simulink library "powerlib"  (Simulink 6.0)
settings: Solver=ode45  SolverMode=SingleTasking  StartTime=0.0  StopTime=10.0  RelTol=1e-3
undefined symbols (not defined in the file or in its folder): com, ctrl1, Da, DiscIntNeverNeededParam, dtha, etat, FA, find_system, Ha, j, Ka, Ki, Kv, q0, Rground, sel, st_a, st_b, st_c, sta, stb, stc, T1, T2, T3, T4
libraries: powerlib_models x30, powerlib x25, simulink_extras x6, powerlib_extras x3, simulink x2
(part 4 of 7)

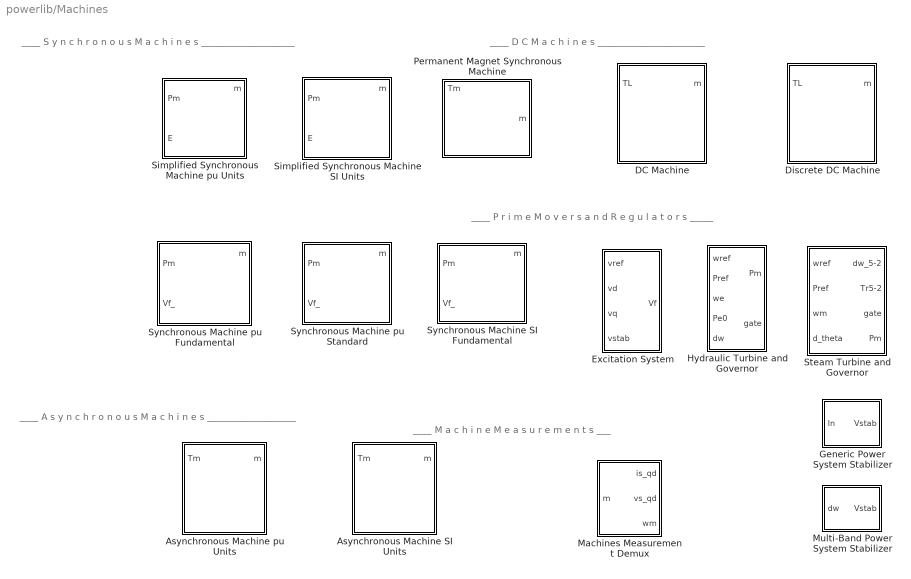
== system powerlib/Machines ==
  note: ____ A s y n c h r o n o u s M a c h i n e s ___________________
  note: ____ M a c h i n e M e a s u r e m e n t s ___
  note: ____ P r i m e M o v e r s a n d R e g u l a t o r s _____
  note: ____ D C M a c h i n e s _______________________
  note: ____ S y n c h r o n o u s M a c h i n e s ____________________
  Asynchronous Machine SI Units : Subsystem  mask(Asynchronous Machine){PresetModel=No, ShowDetailedParameters=on, RotorType=Wound, ReferenceFrame=Rotor, NominalParameters=[3730 460 60], Stator=[1.115 0.005974], Rotor=[1.083 0.005974], Lm=0.2037, Mechanical=[0.02 0.005752 2], InitialConditions=[ 1,0   0,0,0   0,0,0 ], Units=1, LoadFlowParameters=0}
      mask prompts: PresetModel "Preset model:"; ShowDetailedParameters "-----------------  Show detailed parameters -----------------"; RotorType "Rotor type:"; ReferenceFrame "Reference frame:"; NominalParameters "Nominal power, voltage (line-line), and frequency [ Pn(VA),Vn(Vrms),fn(Hz) ]:"; Stator "Stator resistance and inductance[ Rs(ohm)  Lls(H) ]:"; Rotor "Rotor resistance and inductance [ Rr'(ohm)  Llr'(H) ]:"; Lm "Mutual inductance Lm (H):"; Mechanical "Inertia, friction factor and pairs of poles [ J(kg.m^2)  F(N.m.s)  p() ]:"; InitialConditions "Initial conditions"; Units "IOunits"; LoadFlowParameters "Load flow Parameters"
      mask help:
      | Implements a three-phase asynchronous machine (wound rotor or squirrel cage)
      | modeled in the dq rotor reference frame. Stator and rotor windings are connected
      | in wye to an internal neutral point. You can specify initial values for stator and rotor
      | currents or for  the stator current only.
      mask init:
      | block = gcb;
      | ctrl = ReferenceFrame;
      | one_third=1/3; 
      | sqrt3_3=sqrt(3)/3;
      | sqrt3=sqrt(3);
      | switch RotorType
      |     case 1, selWidth=6; elements1=3:6; elements2=1:4;
      |     case 2, selWidth=4; elements1=1:4; elements2=3:4;
      | end
      | powericon('psbloadfunction',block,'gotofrom','Initialize');
      | [NominalParameters,Stator,Rotor,Lm,Mechanical,InitialConditions] = powericon('AsynchronousMachineConvert',NominalParameters,Stator,Rotor,Lm,Mechanical,InitialConditions);	
      | Ts = powericon('AsynchronousMachineInit',block);
      | [p1,p2,p3,p4,p5,p6,p7,p8,p9,p10,p11,p12,p13,p14,p15,p16] = powericon('AsynchronousMachineIcon');
      | [Rs,Lls,Rr,Llr,H,F,p,Laq,Lad,web_psb,Vb,Vb2,ib,ib2,phib2,Nb2,Tb2,phisqo,phisdo,phirqo,phirdo,wmo,tho] = powericon('AsynchronousMachineParam',NominalParameters,Stator,Rotor,Lm,Mechanical,InitialConditions,Units);
      | powericon('AsynchronousMachineCback',block);
      settings: CopyFcn=powericon('psbloadfunction',gcbh,'gotofrom','UpdateGotoTag');
      mask Help: web(psbhelp);
      mask StyleString: popup(No|01:  5 HP   460 V 60Hz 1750 RPM           |02:  10 HP  460 V 60Hz 1760 RPM          |03:  20 HP  460 V 60Hz 1760 RPM          |04:  50 HP  460 V 60Hz 1780 RPM          |05:  100 HP 460 V 60Hz 1780 RPM         |06:  150 HP 460 V 60Hz 1785 RPM         |07:  200 HP 460 V 60Hz 1785 RPM         |08:  5 HP   575 V 60Hz 1750 RPM           |09:  10 HP  575 V 60Hz 1760 RPM          |10:  20 HP  575 V 60Hz 1765 RPM          |11:  50 HP  575 V 60Hz 1775 RPM          |12:  100 HP 575 V 60Hz 1780 RPM         |13:  150 HP 575 V 60Hz 1785 RPM         |14:  200 HP 575 V 60Hz 1785 RPM         |15:  5.4 HP (4KW)   400 V  50Hz 1430 RPM  |16:  10 HP (7.5KW)  400 V 50Hz 1440 RPM |17:  20 HP (15KW)   400 V 50Hz 1460 RPM  |18:  50 HP (37KW)   400 V 50Hz 1480 RPM  |19:  100 HP (75KW)  400 V 50Hz 1484 RPM |20:  150 HP (110KW) 400 V 50Hz 1487 RPM|21:  215 HP (160KW) 400 V 50Hz 1487 RPM),checkbox,popup(Wound|Squirrel-cage),popup(Rotor|Stationary|Synchronous),edit,edit,edit,edit,edit,edit,edit,edit
      mask CallbackString: powericon('AsynchronousMachineCback',gcb,'SI');|powericon('AsynchronousMachineCback',gcb);|powericon('AsynchronousMachineCback',gcb);|||||||||
      mask Display: plot(-55,-30,55,90,p1,p2,p3,p4,p5,p6,p7,p8,p9,p10,p11,p12,p13,p14,p15,p16);color('blue');plot([-30,-10,-10],[70,70,55]);plot([35,10,10],[70,70,55]);
  Asynchronous Machine pu Units : Subsystem  mask(Asynchronous Machine){PresetModel=No, ShowDetailedParameters=on, RotorType=Wound, ReferenceFrame=Rotor, NominalParameters=[3730 460 60], Stator=[0.01965 0.0397], Rotor=[0.01909 0.0397], Lm=1.354, Mechanical=[0.09526 0.05479 2], InitialConditions=[ 1,0   0,0,0   0,0,0 ], Units=0, LoadFlowParameters=0}
      mask prompts: PresetModel "Preset model:"; ShowDetailedParameters "-----------------  Show detailed parameters -----------------"; RotorType "Rotor type:"; ReferenceFrame "Reference frame:"; NominalParameters "Nominal power, voltage (line-line), and frequency  [ Pn(VA),Vn(Vrms),fn(Hz) ]:"; Stator "Stator resistance and inductance  [ Rs,Lls ] (pu):"; Rotor "Rotor resistance and inductance  [ Rr',Llr' ] (pu):"; Lm "Mutual inductance Lm (pu):"; Mechanical "Inertia constant, friction factor and pairs of poles [ H(s) F(pu) p() ]:"; InitialConditions "Initial conditions"; Units "IOunits"; LoadFlowParameters "Load Flow Parameters"
      mask help:
      | Implements a three-phase asynchronous machine (wound rotor or squirrel cage)
      | modeled in the dq rotor reference frame. Stator and rotor windings are connected
      | in wye to an internal neutral point. You can specify initial values for stator and rotor
      | currents or for  the stator current only.
      mask init:
      | block = gcb;
      | ctrl = ReferenceFrame;
      | one_third=1/3; 
      | sqrt3_3=sqrt(3)/3;
      | sqrt3=sqrt(3);
      | switch RotorType
      |     case 1, selWidth=6; elements1=3:6; elements2=1:4;
      |     case 2, selWidth=4; elements1=1:4; elements2=3:4;
      | end
      | Ts = powericon('AsynchronousMachineInit',block);
      | powericon('psbloadfunction',block,'gotofrom','Initialize');
      | [p1,p2,p3,p4,p5,p6,p7,p8,p9,p10,p11,p12,p13,p14,p15,p16] = powericon('AsynchronousMachineIcon');
      | [Rs,Lls,Rr,Llr,H,F,p,Laq,Lad,web_psb,Vb,Vb2,ib,ib2,phib2,Nb2,Tb2,phisqo,phisdo,phirqo,phirdo,wmo,tho] = powericon('AsynchronousMachineParam',NominalParameters,Stator,Rotor,Lm,Mechanical,InitialConditions,Units);
      | powericon('AsynchronousMachineCback',block);
      settings: CopyFcn=powericon('psbloadfunction',gcb,'gotofrom','UpdateGotoTag');
      mask Help: web(psbhelp);
      mask StyleString: popup(No|01:  5 HP   460 V 60Hz 1750 RPM           |02:  10 HP  460 V 60Hz 1760 RPM          |03:  20 HP  460 V 60Hz 1760 RPM          |04:  50 HP  460 V 60Hz 1780 RPM          |05:  100 HP 460 V 60Hz 1780 RPM         |06:  150 HP 460 V 60Hz 1785 RPM         |07:  200 HP 460 V 60Hz 1785 RPM         |08:  5 HP   575 V 60Hz 1750 RPM           |09:  10 HP  575 V 60Hz 1760 RPM          |10:  20 HP  575 V 60Hz 1765 RPM          |11:  50 HP  575 V 60Hz 1775 RPM          |12:  100 HP 575 V 60Hz 1780 RPM         |13:  150 HP 575 V 60Hz 1785 RPM         |14:  200 HP 575 V 60Hz 1785 RPM         |15:  5.4 HP (4KW)   400 V  50Hz 1430 RPM  |16:  10 HP (7.5KW)  400 V 50Hz 1440 RPM |17:  20 HP (15KW)   400 V 50Hz 1460 RPM  |18:  50 HP (37KW)   400 V 50Hz 1480 RPM  |19:  100 HP (75KW)  400 V 50Hz 1484 RPM |20:  150 HP (110KW) 400 V 50Hz 1487 RPM|21:  215 HP (160KW) 400 V 50Hz 1487 RPM),checkbox,popup(Wound|Squirrel-cage),popup(Rotor|Stationary|Synchronous),edit,edit,edit,edit,edit,edit,edit,edit
      mask CallbackString: powericon('AsynchronousMachineCback',gcb,'pu');|powericon('AsynchronousMachineCback',gcb);|powericon('AsynchronousMachineCback',gcb);|||||||||
      mask Display: plot(-55,-30,55,90,p1,p2,p3,p4,p5,p6,p7,p8,p9,p10,p11,p12,p13,p14,p15,p16);color('blue');plot([-30,-10,-10],[70,70,55]);plot([35,10,10],[70,70,55]);
  DC Machine : Subsystem  LoadFcn=find_system(gcs,'FollowLinks', 'on', 'LookUnderMasks', 'all');  mask(DC machine){PresetModel=No, ShowDetailedParameters=on, RLa=[ 0.5  0.01], RLf=[ 240  120], Laf=1.8, J=0.05, Bm=0.02, Tf=0, w0=0}
      mask prompts: PresetModel "Preset  model"; ShowDetailedParameters "-----------------  Show detailed parameters -----------------"; RLa "Armature resistance and inductance [Ra (ohms) La (H) ]"; RLf "Field resistance and inductance [Rf (ohms) Lf (H) ]"; Laf "Field-armature mutual inductance Laf (H) :"; J "Total inertia J (kg.m^2)"; Bm "Viscous friction coefficient Bm (N.m.s)"; Tf "Coulomb friction torque Tf (N.m)"; w0 "Initial speed (rad/s) :"
      mask help: This block implements a separately excited DC machine. Access is provided to the field connections so that the machine can be used as a shunt-connected or a series-connected DC machine.
      mask init:
      | Ra=RLa(1); La=RLa(2);
      | 
      | Rf=RLf(1); Lf=RLf(2);
      mask Help: web(psbhelp)
      mask StyleString: popup(No|01: 5HP 240V 1750RPM Field:300V|02: 5HP 240V 1750RPM Field:150V|03: 5HP 500V 1750RPM Field:300V|04: 10HP 240V 1750RPM Field:300V|05: 10HP 500V 1750RPM Field:300V|06: 20HP 240V 1750RPM Field:300V|07: 20HP 500V 1750RPM Field:300V|08: 30HP 240V 1750RPM Field:300V|09: 30HP 500V 1750RPM Field:300V|10: 40HP 240V 1750RPM Field:300V|11: 40HP 500V 1750RPM Field:300V|12: 50HP 240V 1750RPM Field:300V|13: 50HP 500V 1750RPM Field:300V|14: 75HP 500V 1750RPM Field:300V|15: 100HP 500V 1750RPM Field:300V|16: 125HP 500V 1750RPM Field:300V|17: 150HP 500V 1750RPM Field:300V|18: 175HP 500V 1750RPM Field:300V|19: 200HP 440V 1184RPM Field:310V|20: 200HP 500V 1750RPM Field:150V|21: 200HP 500V 1750RPM Field:300V|22: 225HP 500V 1750RPM Field:300V|23: 250HP 500V 1750RPM Field:300V),checkbox,edit,edit,edit,edit,edit,edit,edit
      mask CallbackString: powericon('DCMachineCback',gcb,'Continuous');|powericon('DCMachineCback',gcb,'Continuous');|||||||
      mask Display:
      | plot(-80,-80,80,80,[0,9,18,24,29,30,29,24,18,9,0,-9,-18,-24,-29,-30,-29,-24,-18,-9,0],[30,29,24,18,9,0,-9,-18,-24,-29,-30,-29,-24,-18,-9,0,9,18,24,29,30],[-29,-35,-35,-29],[-8,-8,8,8],[29,35,35,29],[-8,-8,8,8],[-35,-55],[0,0],[35,55],[0,0],[-78,-50,-50,-49,-45,-39,-33,-26,-21,-18,-17,-19,-22,-22,-26,-27,-25,-22,-16,-9,-3,2,6,6,4,1,1,-3,-4,-2,2,7,14,20,26,29,30,28,24,24,21,20,21,25,31,37,44,49,50,50,50,78]*.7,[58,58,57.2,49.2,42.8,38.8,38,39.6,44.4,51.6,59.6,67.6,72.4,72.4,65.2,57.2,49.2,42.8,38.8,38,39.6,44.4,51.6,59.6,67.6,72.4,72.4,65.2,57.2,49.2,42.8,38.8,38,39.6,44.4,51.6,59.6,67.6,72.4,72.4,65.2,57.2,49.2,42.8,38.8,38,39.6,44.4,51.6,58,58,58]*.6-85 );
      | 
      | disp('dc')
      | 
      | color('blue');
      | 
      | plot([-50,-10,-10],[50,50,30]);
      | 
      | plot([50,10,10],[50,50,30]);
  Discrete DC Machine : Subsystem  LoadFcn=find_system(gcs,'FollowLinks', 'on', 'LookUnderMasks', 'all');  mask(Discrete DC machine){PresetModel=No, ShowDetailedParameters=on, RLa=[0.5  0.01], RLf=[240  120], Laf=1.8, J=0.05, Bm=0.02, Tf=0, w0=0, Ts=50e-6}
      mask prompts: PresetModel "Preset  model"; ShowDetailedParameters "-----------------  Show detailed parameters -----------------"; RLa "Armature resistance and inductance [Ra (ohms) La (H) ]"; RLf "Field resistance and inductance [Rf (ohms) Lf (H) ]"; Laf "Field-armature mutual inductance Laf (H) :"; J "Total inertia J (kg.m^2)"; Bm "Viscous friction coefficient Bm (N.m.s)"; Tf "Coulomb friction torque Tf (N.m)"; w0 "Initial speed (rad/s) :"; Ts "Sample Time"
      mask help: This block implements a separately excited DC machine. Access is provided to the field connections so that the machine can be used as a shunt-connected or a series-connected DC machine.
      mask init:
      | Ra=RLa(1); La=RLa(2);
      | 
      | Rf=RLf(1); Lf=RLf(2);
      settings: AttributesFormatString=\n
      mask Help: web(psbhelp)
      mask StyleString: popup(No|01: 5HP 240V 1750RPM Field:300V|02: 5HP 240V 1750RPM Field:150V|03: 5HP 500V 1750RPM Field:300V|04: 10HP 240V 1750RPM Field:300V|05: 10HP 500V 1750RPM Field:300V|06: 20HP 240V 1750RPM Field:300V|07: 20HP 500V 1750RPM Field:300V|08: 30HP 240V 1750RPM Field:300V|09: 30HP 500V 1750RPM Field:300V|10: 40HP 240V 1750RPM Field:300V|11: 40HP 500V 1750RPM Field:300V|12: 50HP 240V 1750RPM Field:300V|13: 50HP 500V 1750RPM Field:300V|14: 75HP 500V 1750RPM Field:300V|15: 100HP 500V 1750RPM Field:300V|16: 125HP 500V 1750RPM Field:300V|17: 150HP 500V 1750RPM Field:300V|18: 175HP 500V 1750RPM Field:300V|19: 200HP 440V 1184RPM Field:310V|20: 200HP 500V 1750RPM Field:150V|21: 200HP 500V 1750RPM Field:300V|22: 225HP 500V 1750RPM Field:300V|23: 250HP 500V 1750RPM Field:300V),checkbox,edit,edit,edit,edit,edit,edit,edit,edit
      mask CallbackString: powericon('DCMachineCback',gcb,'Discrete');|powericon('DCMachineCback',gcb,'Discrete');||||||||
      mask Display:
      | plot(-80,-80,80,80,[0,9,18,24,29,30,29,24,18,9,0,-9,-18,-24,-29,-30,-29,-24,-18,-9,0],[30,29,24,18,9,0,-9,-18,-24,-29,-30,-29,-24,-18,-9,0,9,18,24,29,30],[-29,-35,-35,-29],[-8,-8,8,8],[29,35,35,29],[-8,-8,8,8],[-35,-55],[0,0],[35,55],[0,0],[-78,-50,-50,-49,-45,-39,-33,-26,-21,-18,-17,-19,-22,-22,-26,-27,-25,-22,-16,-9,-3,2,6,6,4,1,1,-3,-4,-2,2,7,14,20,26,29,30,28,24,24,21,20,21,25,31,37,44,49,50,50,50,78]*.7,[58,58,57.2,49.2,42.8,38.8,38,39.6,44.4,51.6,59.6,67.6,72.4,72.4,65.2,57.2,49.2,42.8,38.8,38,39.6,44.4,51.6,59.6,67.6,72.4,72.4,65.2,57.2,49.2,42.8,38.8,38,39.6,44.4,51.6,59.6,67.6,72.4,72.4,65.2,57.2,49.2,42.8,38.8,38,39.6,44.4,51.6,58,58,58]*.6-85 );
      | 
      | disp('dc')
      | 
      | color('blue');
      | 
      | plot([-50,-10,-10],[50,50,30]);
      | 
      | plot([50,10,10],[50,50,30]);
  Excitation System : Subsystem  mask(Excitation System){tr=20e-3, reg=[ 300, 0.001 ], exc=[ 1, 0 ], tgr=[ 0, 0 ], damp=[ 0.001, 0.1 ], sat=[ 0, 0 ], lim=[ -11.5, 11.5, 0 ], v0=[1.0  1.28]}
      mask prompts: tr "Low-pass filter time constant Tr(s):"; reg "Regulator gain and time constant [ Ka()  Ta(s) ]:"; exc "Exciter  [ Ke()  Te(s) ]:"; tgr "Transient gain reduction [ Tb(s)  Tc(s) ]:"; damp "Damping filter gain and time constant  [ Kf()  Tf(s)  ]:"; sat "Field saturation parameters [ A, B ]:"; lim "Regulator output limits and gain [ Efmin, Efmax (p.u.), Kp() ]:"; v0 "Initial values of terminal voltage  and field voltage [ Vt0 (pu) Vf0(pu) ] :"
      mask help:
      | Implements an IEEE type 1 synchronous machine voltage regulator combined
      | to an exciter.
      |
      | The output of the block is the field voltage vfd, in p.u.,  to be applied to the Vf
      | Simulink input of a Synchronous Machine block.
      |
      | Connect the Vd and Vq measurements signals of the Synchronous Machine block
      | (signals 9 and 10)  to  the Vd and Vq inputs of the Excitation System block.
      mask init:
      | ka=reg(1);ta=reg(2);ke=exc(1);te=exc(2);tb=tgr(1);tc=tgr(2);kf=damp(1);tf=damp(2);efmin=lim(1);efmax=lim(2);a=sat(1);b=sat(2);kp=lim(3);
      | powericon('psbcallbacks',gcb,'Excitationsystem',1);
      mask Help: web(psbhelp);
  Generic Power System Stabilizer : Subsystem  mask(Generic Power System Stabilizer){Tsensor=30e-3, K=20, Twashout=2, Tleadlag1=[50e-3 20e-3], Tleadlag2=[3 5.4], VSlimits=[-0.15 0.15], Vinit=0, Plot_On=off, MagdB_On=on, FreqRange=logspace(-2,2,500)}
      mask prompts: Tsensor "Sensor time constant:"; K "Gain:"; Twashout "Wash-out time constant:"; Tleadlag1 "Lead-lag #1 time constants: [ Tnum Tden ]"; Tleadlag2 "Leag-lag #2 time constants: [ Tnum Tden ]"; VSlimits "Output limits: [ VSmin VSmax ]"; Vinit "Initial input:"; Plot_On "Plot frequency response"; MagdB_On "Magnitude in dB"; FreqRange "Frequency range (Hz):"
      mask help:
      | This block implements a generic Power System Stabilizer (PSS). It consists of a
      | low-pass filter, a general gain, a washout high-pass filter, a phase-compensation
      | system, and an output limiter.
      |
      | The input is the synchronous machine speed deviation with respect to nominal
      | (dw in pu) or the acceleration power (Pa=Pm-Pe in pu).
      |
      | The output is the stabilization voltage, in p.u.
      mask init:
      | powericon('psbcallbacks',gcb,'PSS',1);
      | T1n=Tleadlag1(1);
      | T1d=Tleadlag1(2);
      | T2n=Tleadlag2(1);
      | T2d=Tleadlag2(2);
      | %
      | if Plot_On==1,
      | % Compute global system (sysG):
      | numS=[1];
      | denS=[Tsensor 1];
      | sysS=tf(numS,denS);
      | numW=[Twashout 0];
      | denW=[Twashout 1];
      | sysW=tf(numW,denW);
      | numL1=[T1n 1];
      | denL1=[T1d 1];
      | sysL1=tf(numL1,denL1);
      | numL2=[T2n 1];
      | denL2=[T2d 1];
      | sysL2=tf(numL2,denL2);
      | sysG=sysS*K*sysW*sysL1*sysL2;
      | %
      | % Plot response:
      | w=2*pi*FreqRange;
      | [Mag,Pha]=bode(sysG,w);
      | subplot(2,1,1)
      | if  MagdB_On==1,
      | Y= 20*log10(squeeze(Mag)) ;
      | strLabel='dB';
      | else
      | Y=squeeze(Mag);
      | strLabel='pu/pu';
      | end
      | %
      | semilogx(FreqRange,Y)
      | ylabel(strLabel);grid;
      | title('PSS Frequency Response');
      | subplot(2,1,2);
      | semilogx(FreqRange,rem(squeeze(Pha),360))
      | ylabel('Degrees');grid;
      | xlabel('Frequency (Hz)');
      | end
      mask Help: web(psbhelp)
      mask CallbackString: |||||||powericon('psbcallbacks',gcbh,'PSSmodel');||
  Hydraulic Turbine and Governor : Subsystem  mask(Hydraulic Turbine and Governor){sm=[ 10/3  0.07 ], gate=[  0.01  0.97518  -0.1  0.1 ], reg=[  0.05  1.163  0.105  0  0.01  ], hyd=[  0  2.67  ], dref=0, po=0.7516}
      mask prompts: sm "Servo-motor [ Ka()  Ta(sec) ]:"; gate "Gate opening limits [ gmin,gmax(pu)    vgmin,vgmax(pu/s) ]:"; reg "Permanent droop and regulator  [ Rp() Kp() Ki() Kd() Td(s) ]:"; hyd "Hydraulic turbine [ beta()  Tw(sec) ]:"; dref "Droop reference (0=power error, 1=gate opening):"; po "Initial mechanical power (pu):"
      mask help: Implements a hydraulic turbine combined to a PID governor system.
      mask init:
      | ka=sm(1);ta=sm(2);gmin=gate(1);gmax=gate(2);vgmin=gate(3);vgmax=gate(4);Rp=reg(1);kp=reg(2);ki=reg(3);kd=reg(4);td=reg(5);beta=hyd(1);tw=hyd(2);go=po*(gmax-gmin);
      | powericon('psbcallbacks',gcb,'HTGsystem',1);
      mask Help: web(psbhelp);
  Machines Measurement Demux : Subsystem  mask(Machine measurements){machType=Synchronous, ssm1=on, ssm2=on, ssm3=on, ssm4=on, ssm5=on, ssm6=on, sm1=off, sm2=on, sm3=off, sm4=off, sm5=off, sm6=on, sm7=off, sm8=on, sm9=off, sm10=off, sm11=off, sm115=off, sm12=off, sm13=off, sm14=off, asm1=on, asm2=on, asm3=on, asm4=on, asm5=on, asm6=on, asm7=on, asm8=on, asm9=on, asm10=on, asm11=on, pmsm1=on, pmsm2=on, pmsm3=on, pmsm4=on, pmsm5=on, pmsm6=on, lastType=1}
      mask prompts: machType "Machine type:"; ssm1 "Line currents          [ isa  isb  isc ]"; ssm2 "Terminal voltages   [ va  vb  vc ]"; ssm3 "Internal voltages     [ ea  eb  ec ]"; ssm4 "Rotor angle            [ thetam ]   rad"; ssm5 "Rotor speed           [ wm ]"; ssm6 "Electrical power     [ Pe ]"; sm1 "Stator currents                  [ isa  isb  isc ]"; sm2 "Stator currents                  [ iq  id ]"; sm3 "Field current                      [ ifd ]"; sm4 "Damper winding currents   [ ikq1  ikq2  ikd ]"; sm5 "Mutual fluxes                     [ phim_q   phim_d ]"; sm6 "Stator voltages                  [ vs_q   vs_d ]"; sm7 "Rotor angle deviation        [ d_theta ]   rad"; sm8 "Rotor speed                       [ wm ]"; sm9 "Electrical power                 [ Pe ]"; sm10 "Rotor speed deviation       [ dw ]"; sm11 "Rotor mechanical angle     [ theta ]   deg"; sm115 "Electromagnetic torque     [ Te ]"; sm12 "Load angle                         [ Delta ]   deg"; sm13 "Output active power          [ Peo ]"; sm14 "Output reactive power       [ Qeo ]"; asm1 "Rotor currents    [ ira  irb  irc ]"; asm2 "Rotor currents    [ ir_q   ir_d  ]"; asm3 "Rotor fluxes       [ phir_q   phir_d ]"; asm4 "Rotor voltages   [ vr_q   vr_d ]"; asm5 "Stator currents   [ ia  ib  ic ]"; asm6 "Stator currents   [ is_q   is_d ]"; asm7 "Stator fluxes      [ phis_q  phis_d ]"; asm8 "Stator voltages   [ vs_q  vs_d ]"; asm9 "Rotor speed       [ wm ]"; asm10 "Electromagnetic torque  [Te ]"; asm11 "Rotor angle        [ thetam ]  rad"; pmsm1 "Stator currents   [ ia, ib, ic ]  A"; pmsm2 "stator currents    [ is_q   is_d ]  A"; pmsm3 "Stator voltages   [ vs_q   vs_d ]   V"; pmsm4 "Rotor speed       [ wm ]   rad/s"; pmsm5 "Rotor angle        [ thetam ]  rad"; pmsm6 "Electromagnetic torque  [Te ]  N.m"
      mask help: Split specified signals of various machine models measurement output vector into separate signals.
      mask init:
      | t = powericon('Machines Demux Model',gcb);
      mask Help: web(psbhelp);
      mask StyleString: popup(Simplified synchronous|Synchronous|Asynchronous|Permanent magnet synchronous),checkbox,checkbox,checkbox,checkbox,checkbox,checkbox,checkbox,checkbox,checkbox,checkbox,checkbox,checkbox,checkbox,checkbox,checkbox,checkbox,checkbox,checkbox,checkbox,checkbox,checkbox,checkbox,checkbox,checkbox,checkbox,checkbox,checkbox,checkbox,checkbox,checkbox,checkbox,checkbox,checkbox,checkbox,checkbox,checkbox,checkbox,checkbox,edit
      mask CallbackString: powericon('psbcbmachdemux',gcb);|||||||||||||||||||||||||||||||||||||||
      mask Display: plot([0 0],[t t])
  Multi-Band Power System Stabilizer : Subsystem  mask(Multi-Band Power System Stabilizer ){OperationMode=Simplified settings, Kg=1.0, GL=[0.2 20], GI=[0.9 25], GH=[12.0 145], GLd=[66 66 9.4], TcLF=[1.667 2 0 0 0 0 2 2.4 0 0 0 0 1 1], GId=[66 66 47.6], TcIF=[1 1 0.25 0.3 0 0 1 1 0.3 0.36 0 0 0 0], GHd=[66 66 233], TcHF=[0.01 0.012 0 0 0 0  0.012 0.0144 0 0 0 0 1 1], LIM=[.075 .15 .15 .15], Plot_On=off, MagdB_On=off, FreqRange=logspace(-2,2,500)}
      mask prompts: OperationMode "Mode of operation:"; Kg "Global gain:"; GL "Low frequency band: [ FL(Hz), KL ]"; GI "Intermediate frequency band: [ FI(Hz), KI ]"; GH "High frequency band: [ FH(Hz), KH ]"; GLd "Low frequency gains: [ KL1, KL2, KL ]"; TcLF "Low frequency  time constants (s):"; GId "Intermediate frequency gains: [ KI1, KI2, KI ]"; TcIF "Intermediate frequency time constants (s):"; GHd "High frequency gains: [ KH1, KH2, KH ]"; TcHF "High frequency time constants (s):"; LIM "Signals Limits(VLmax,VImax,VHmax,VSmax)"; Plot_On "Plot frequency response"; MagdB_On "Magnitude in dB"; FreqRange "Frequency range (Hz):"
      mask help:
      | This block implements a Multi-band Power System Stabilizer (MB-PSS). Two operation modes are available: Detailed setting and simplified setting (IEEE Std 421.5).
      |
      | When "Detailed settings" is used, the low(L)-, intermediate(I)- and high(H)-frequency time constants must be given in the following order:
      | Tx1 to Tx12 followed by Kx11 and Kx17 (where x=L, I or H).
      mask init:
      | powericon('psbcallbacks',gcb,'MBPSS',1);
      | Detailed=0;
      | if OperationMode==2,
      | Detailed=1;
      | Kg=1;
      | KL1=GLd(1);KL2=GLd(:,2);KL=GLd(3);
      | TL1=TcLF(1);TL2=TcLF(2);TL3=TcLF(3);TL4=TcLF(4);
      | TL5=TcLF(5);TL6=TcLF(6);TL7=TcLF(7);TL8=TcLF(8);
      | TL9=TcLF(9);TL10=TcLF(10);TL11=TcLF(11);TL12=TcLF(12);
      | KL11=TcLF(13);KL17=TcLF(14);
      | KI1=GId(1);KI2=GId(:,2);KI=GId(3);
      | TI1=TcIF(1);TI2=TcIF(2);TI3=TcIF(3);TI4=TcIF(4);
      | TI5=TcIF(5);TI6=TcIF(6);TI7=TcIF(7);TI8=TcIF(8);
      | TI9=TcIF(9);TI10=TcIF(10);TI11=TcIF(11);TI12=TcIF(12);
      | KI11=TcIF(13);KI17=TcIF(14);
      | KH1=GHd(1);KH2=GHd(:,2);KH=GHd(3);
      | TH1=TcHF(1);TH2=TcHF(2);TH3=TcHF(3);TH4=TcHF(4);
      | TH5=TcHF(5);TH6=TcHF(6);TH7=TcHF(7);TH8=TcHF(8);
      | TH9=TcHF(9);TH10=TcHF(10);TH11=TcHF(11);TH12=TcHF(12);
      | KH11=TcHF(13);KH17=TcHF(14);
      | else
      | %
      | R=1.2;K=(R*R+R)/(R*R-2*R+1);KL1=K;KL2=K;KI1=K;KI2=K;KH1=K;KH2=K;
      | TL2=1/(2*pi*GL(1)*sqrt(R));KL=GL(2);TL1=TL2/R;TL7=TL2;TL8=TL7*R;
      | %
      | TI2=1/(2*pi*GI(1)*sqrt(R));KI=GI(2);TI1=TI2/R;TI7=TI2;TI8=TI7*R;
      | TH2=1/(2*pi*GH(1)*sqrt(R));KH=GH(2);TH1=TH2/R;TH7=TH2;TH8=TH7*R;
      | %
      | TL3=0;TL4=0;TL5=0;TL6=0;TL9=0;TL10=0;TL11=0;TL12=0;
      | TI3=0;TI4=0;TI5=0;TI6=0;TI9=0;TI10=0;TI11=0;TI12=0;
      | TH3=0;TH4=0;TH5=0;TH6=0;TH9=0;TH10=0;TH11=0;TH12=0;
      | KL11=1;KL17=1;KI11=1;KI17=1;KH11=1;KH17=1;
      | end
      | LIM_VL=LIM(1);LIM_VI=LIM(2);LIM_VH=LIM(3);LIM_VS=LIM(4);
      | %
      | % LF Transfer function
      | numLF1=[TL1 KL11];
      | denLF1=[TL2 1];
      | sysLF1=tf(numLF1,denLF1);
      | numLF2=[TL3 1];
      | denLF2=[TL4 1];
      | sysLF2=tf(numLF2,denLF2);
      | numLF3=[TL5 1];
      | denLF3=[TL6 1];
      | sysLF3=tf(numLF3,denLF3);
      | numLF4=[TL7 KL17];
      | denLF4=[TL8 1];
      | sysLF4=tf(numLF4,denLF4);
      | numLF5=[TL9 1];
      | denLF5=[TL10 1];
      | sysLF5=tf(numLF5,denLF5);
      | numLF6=[TL11 1];
      | denLF6=[TL12 1];
      | sysLF6=tf(numLF6,denLF6);
      | %
      | sysLF=Kg*KL*((KL1*sysLF1*sysLF2*sysLF3) - (KL2*sysLF4*sysLF5*sysLF6));
      | %
      | %
      | % IF transfer function
      | numIF1=[TI1 KI11];
      | denIF1=[TI2 1];
      | sysIF1=tf(numIF1,denIF1);
      | numIF2=[TI3 1];
      | denIF2=[TI4 1];
      | sysIF2=tf(numIF2,denIF2);
      | numIF3=[TI5 1];
      | denIF3=[TI6 1];
      | sysIF3=tf(numIF3,denIF3);
      | numIF4=[TI7 KI17];
      | denIF4=[TI8 1];
      | sysIF4=tf(numIF4,denIF4);
      | numIF5=[TI9 1];
      | denIF5=[TI10 1];
      | sysIF5=tf(numIF5,denIF5);
      | numIF6=[TI11 1];
      | denIF6=[TI12 1];
      | sysIF6=tf(numIF6,denIF6);
      | %
      | sysIF=Kg*KI*((KI1*sysIF1*sysIF2*sysIF3) - (KI2*sysIF4*sysIF5*sysIF6));
      | %
      | %
      | % HF transfer function
      | numHF1=[TH1 KH11];
      | denHF1=[TH2 1];
      | sysHF1=tf(numHF1,denHF1);
      | numHF2=[TH3 1];
      | denHF2=[TH4 1];
      | sysHF2=tf(numHF2,denHF2);
      | numHF3=[TH5 1];
      | denHF3=[TH6 1];
      | sysHF3=tf(numHF3,denHF3);
      | numHF4=[TH7 KH17];
      | denHF4=[TH8 1];
      | sysHF4=tf(numHF4,denHF4);
      | numHF5=[TH9 1];
      | denHF5=[TH10 1];
      | sysHF5=tf(numHF5,denHF5);
      | numHF6=[TH11 1];
      | denHF6=[TH12 1];
      | sysHF6=tf(numHF6,denHF6);
      | %
      | sysHF=Kg*KH*((KH1*sysHF1*sysHF2*sysHF3) - (KH2*sysHF4*sysHF5*sysHF6));
      | %
      | %
      | % Input filter LIF
      | numLIFin=[1.759e-3 1];
      | denLIFin=[1.2739e-4 1.7823e-2 1];
      | sysLIFin=tf(numLIFin,denLIFin);
      | % Input filter HF
      | numHFin=[80 0 0];
      | denHFin=[1 82 161 80];
      | sysHFin=tf(numHFin,denHFin);
      | %
      | % Global transfer function:
      | sysL=sysLIFin*sysLF;
      | sysI=sysLIFin*sysIF;
      | sysH=sysHFin*sysHF;
      | sysG=sysL+sysI + sysH;
      | %
      | % Plot frequency response:
      | if Plot_On==1,
      |     w=2*pi*FreqRange;
      |     [MagL,PhaseL]=bode(sysL,w);
      |     [MagI,PhaseI]=bode(sysI,w);
      |     [MagH,PhaseH]=bode(sysH,w);
      |     [MagG,PhaseG]=bode(sysG,w);
      |     subplot(2,1,1)
      |      if  MagdB_On==1,
      |         YL= 20*log10(squeeze(MagL)) ;
      |         YI= 20*log10(squeeze(MagI)) ;
      |         YH= 20*log10(squeeze(MagH)) ;
      |         YG= 20*log10(squeeze(MagG)) ;
      |          strLabel='dB';
      | else
      | YL=squeeze(MagL);
      | YI=squeeze(MagI);
      | YH=squeeze(MagH);
      | YG=squeeze(MagG);
      | strLabel='pu/pu';
      | end
      | semilogx(FreqRange,YL,'m',FreqRange,YI,'g',FreqRange,YH,'b',FreqRange,YG,'r')
      | ylabel(strLabel);grid;
      | legend('LF band','IF band','HF band','Global',2);
      | title('PSS Frequency Response');
      |  subplot(2,1,2);
      | semilogx(FreqRange,rem(squeeze(PhaseL),360),'m',FreqRange,rem(squeeze(PhaseI),360),'g',FreqRange,rem(squeeze(PhaseH),360),'b',FreqRange,rem(squeeze(PhaseG),360),'r');
      | ylabel('Degrees');grid;
      | xlabel('Frequency (Hz)');
      | end
      settings: CopyFcn=powericon('psbcallbacks',gcb,'MBPSS',2);
      mask Help: web(psbhelp)
      mask StyleString: popup(Simplified settings|Detailed settings),edit,edit,edit,edit,edit,edit,edit,edit,edit,edit,edit,checkbox,checkbox,edit
      mask CallbackString: powericon('psbcallbacks',gcb,'MBPSSmodel',1);||||||||||||parametres=get_param(gcb,'MaskValues');p1=parametres{1};p13=parametres{13};if strcmp(p1,'Detailed settings');param2='off';param3='off';param4='off';param5='off';param6='on';param7='on';param8='on';param9='on';param10='on';param11='on';else;param2='on';param3='on';param4='on';param5='on';param6='off';param7='off';param8='off';param9='off';param10='off';param11='off';end;if strcmp(p13,'on');param14='on';param15='on';else;param14='off';param15='off';end;visible={'on',param2,param3,param4,param5,param6,param7,param8,param9,param10,param11,'on','on',param14,param15};set_param(gcb,'MaskVisibilities',visible)||
  Permanent Magnet Synchronous Machine : Subsystem  mask(Permanent Magnet Synchronous Machine){PresetModel=No, ShowDetailedParameters=on, Resistance=2.8750, Inductances=[8.5e-3, 8.5e-3], Flux=0.175, Mechanical=[ 0.8e-3, 0,  4 ]}
      mask prompts: PresetModel "Preset model:"; ShowDetailedParameters "-----------------  Show detailed parameters -----------------"; Resistance "Resistance R(ohm):"; Inductances "Inductances [ Ld(H) Lq(H) ]:"; Flux "Flux induced by magnets (Wb):"; Mechanical "Inertia, friction factor and pairs of poles [ J(kg.m^2)  F(N.m.s)  p() ]:"
      mask help:
      | Implements a 3-phase permanent magnet synchronous machine with sinusoidal flux distribution. The machine is modelled in the dq rotor reference frame. Stator windings are connected in wye to an internal neutral point.
      |
      | Tm:  Mechanical torque, in N.m. Tm > 0 for motor mode, Tm < 0 for generator mode.
      |
      | The preset models are listed by : Rated torque (Nm) @ rated speed (RPM) and maximum bus voltage (Vdc), continuous stall torque (Nm)
      mask init:
      | block = gcb;
      | Ts = powericon('PMSynchronousMachineInit',block);
      | powericon('psbloadfunction',block,'gotofrom','Initialize');
      | [circl1,circl2,a1,a2,b1,b2,c1,c2,d1,d2,n1,n2,s1,s2] = powericon('PMSynchronousMachineIcon');
      | Ld=Inductances(1);
      | Lq=Inductances(2);
      | J=Mechanical(1);
      | F=Mechanical(2);
      | p=Mechanical(3);
      | R=Resistance;
      | sqrt3=sqrt(3);
      | one_third=1/3;
      settings: CopyFcn=powericon('psbloadfunction',gcb,'gotofrom','UpdateGotoTag');
      mask Help: web(psbhelp);
      mask StyleString: popup(No|01:  0.8 Nm 300 Vdc 3000 RPM - 0.8 Nm|02:  1.7 Nm 300 Vdc 3750 RPM - 1.7 Nm|03:  2.8 Nm 300 Vdc 4250 RPM - 3.2 Nm|04:  6 Nm 300 Vdc 4500 RPM - 6 Nm|05:  8 Nm 300 Vdc 2000 RPM - 10 Nm|06:  10 Nm 300 Vdc 2300 RPM - 14.2 Nm|07:  20 Nm 300 Vdc 2200 RPM - 33.9 Nm|08:  24 Nm 300 Vdc 2300 RPM - 41.4 Nm|09:  7.14 Nm 560 Vdc 5000 RPM - 8.3 Nm|10:  7.71 Nm 560 Vdc 5000 RPM - 10.2 Nm|11:  26.13 Nm 560 Vdc 3000 RPM - 27.3 Nm|12:  35.17 Nm 560 Vdc 3000 RPM - 37.4 Nm|13:  42.09 Nm 560 Vdc 3000 RPM - 45.6 Nm|14:  67.27 Nm 560 Vdc 1700 RPM - 70.2 Nm|15:  87.75 Nm 560 Vdc 3000 RPM - 97.96 Nm|16:  111 Nm 560 Vdc 3000 RPM - 126 Nm),checkbox,edit,edit,edit,edit
      mask CallbackString: powericon('PMSynchronousMachineCback',gcb);|powericon('PMSynchronousMachineCback',gcb);||||
      mask Display:
      | plot(-70,-20,55,80,circl1,circl2,a1,a2,b1,b2,c1,c2,d1,d2,n1,n2,s1,s2);
      | color('blue')
      | plot([-40,0,0],[70,70,52])
  Simplified Synchronous Machine SI Units : Subsystem  mask(Simplified Synchronous Machine){ConnectionType=3-wire Y, NominalParameters=[187e6 13800 60], Mechanical=[3.895e6 0 20], InternalRL=[0.0204  0.8104e-3], InitialConditions=[ 0,0   0,0,0   0,0,0 ], Units=1, LoadFlowParameters=[1,0,0,0,0]}
      mask prompts: ConnectionType "Connection type:"; NominalParameters "Nom. power, L-L volt., and freq. [ Pn(VA) Vn(Vrms) fn(Hz) ]:"; Mechanical "Inertia, damping factor and pairs of poles [J(kg.m^2) Kd(pu_T/pu_w) p()]"; InternalRL "Internal impedance [ R(ohm)  L(H) ]:"; InitialConditions "Init. cond. [ dw(%)  th(deg)  ia,ib,ic(A)  pha,phb,phc(deg) ]:"; Units "iounits"; LoadFlowParameters "Load Flow Parameters"
      mask help:
      | Implements a 3-phase simplified synchronous machine. Machine is modelled as an internal voltage behind a R-L impedance. Stator windings are connected in wye to an internal neutral point.
      |
      | Pm:  Mechanical power supplied to the machine, in Watts. Pm>0 for generator mode, Pm<0 for motor mode.
      |
      | E:  RMS value of phase-to-phase internal voltage, in volts.
      mask init:
      | block = gcb;
      | [NominalParameters,Mechanical,InternalRL,InitialConditions] = powericon('SimplifiedSynchronousMachineConvert',NominalParameters,Mechanical,InternalRL,InitialConditions);
      | powericon('psbloadfunction',block,'gotofrom','Initialize');
      | powericon('SimplifiedSynchronousMachineCback',block);
      | Ts = powericon('SimplifiedSynchronousMachineInit',block);
      | circl1=[0,9,18,24,29,30,29,24,18,9,0,-9,-18,-24,-29,-30,-29,-24,-18,-9,0]*1.2;
      | circl2=[30,29,24,18,9,0,-9,-18,-24,-29,-30,-29,-24,-18,-9,0,9,18,24,29,30]*1.2;
      | i1 = [0,-9,-18,-24,-16,-16,-24,-18,-9,0,9,18,24,16,16,24,18,9,0];
      | i2 = [-30,-29,-24,-18,-18,18,18,24,29,30,29,24,18,18,-18,-18,-24,-29,-30]+15;
      | circl2=circl2+15;
      | a1 = [23,48];
      | a2 = [27,27]+15;
      | b1 = [36,48];
      | b2 = [15,15];
      | c1 = [23,48];
      | c2 = [-27,-27]+15;
      | d1 = [-36,-45,-45,60];
      | d2 = [0,0,-50,-50];
      | x9=0;
      | 
      | [Pb,Nb,Vb,Vb2,Vb3,ib,ib2,web_psb,H,Kd,p,pi23,R,L,io,dwo,tho]=powericon('SimplifiedSynchronousMachineParam',NominalParameters,Mechanical,InternalRL,InitialConditions,Units);
      | if ConnectionType==1,sel=1:2; else sel=1:3; end
      | 
      | % phasor model:
      | Id1o=InitialConditions(3)*cos(InitialConditions(6)*pi/180);
      | Iq1o=InitialConditions(3)*sin(InitialConditions(6)*pi/180);
      settings: CopyFcn=powericon('psbloadfunction',gcb,'gotofrom','UpdateGotoTag');
      mask Help: web(psbhelp);
      mask StyleString: popup(3-wire Y|4-wire Y),edit,edit,edit,edit,edit,edit
      mask CallbackString: powericon('SimplifiedSynchronousMachineCback',gcb);||||||
      mask Display: plot(-60,-10,60,80,circl1,circl2,a1,a2,b1,b2,c1,c2);disp('\nSSM');color('blue');plot([0,0,40],[50,68,68]);plot([-35,-25],[50,40]);plot([-45,-35],[0,0])
  Simplified Synchronous Machine pu Units : Subsystem  mask(Simplified Synchronous Machine){ConnectionType=3-wire Y, NominalParameters=[187e6 13800 60], Mechanical=[3.7 0 20], InternalRL=[0.02  0.3], InitialConditions=[ 0,0   0,0,0   0,0,0 ], Units=0, LoadFlowParameters=[1,0,0,0,0]}
      mask prompts: ConnectionType "Connection type:"; NominalParameters "Nom. power, L-L volt., and freq. [ Pn(VA) Vn(Vrms) fn(Hz) ]:"; Mechanical "Inertia, damping factor and pairs of poles [H(sec) Kd(pu_T/pu_w) p()]"; InternalRL "Internal impedance [ R(pu)  X(pu) ]:"; InitialConditions "Init. cond. [ dw(%)  th(deg)  ia,ib,ic(pu)  pha,phb,phc(deg) ]:"; Units "iounits"; LoadFlowParameters "Load Flow Parameters"
      mask help:
      | Implements a 3-phase simplified synchronous machine. Machine is modeled
      | as an internal voltage behind a R-L impedance. Stator windings are connected
      | in wye to an internal neutral point.
      mask init:
      | block = gcb;
      | powericon('SimplifiedSynchronousMachineCback',block);
      | Ts = powericon('SimplifiedSynchronousMachineInit',block);
      | powericon('psbloadfunction',block,'gotofrom','Initialize');
      | circl1=[0,9,18,24,29,30,29,24,18,9,0,-9,-18,-24,-29,-30,-29,-24,-18,-9,0]*1.2;
      | circl2=[30,29,24,18,9,0,-9,-18,-24,-29,-30,-29,-24,-18,-9,0,9,18,24,29,30]*1.2;
      | i1 = [0,-9,-18,-24,-16,-16,-24,-18,-9,0,9,18,24,16,16,24,18,9,0];
      | i2 = [-30,-29,-24,-18,-18,18,18,24,29,30,29,24,18,18,-18,-18,-24,-29,-30]+15;
      | circl2=circl2+15;
      | a1 = [23,48];
      | a2 = [27,27]+15;
      | b1 = [36,48];
      | b2 = [15,15];
      | c1 = [23,48];
      | c2 = [-27,-27]+15;
      | d1 = [-36,-45,-45,60];
      | d2 = [0,0,-50,-50];
      | x9=0;
      | 
      | [Pb,Nb,Vb,Vb2,Vb3,ib,ib2,web_psb,H,Kd,p,pi23,R,L,io,dwo,tho]=powericon('SimplifiedSynchronousMachineParam',NominalParameters,Mechanical,InternalRL,InitialConditions,Units);
      | if ConnectionType==1,sel=1:2; else sel=1:3; end
      | Id1o=InitialConditions(3)*cos(InitialConditions(6)*pi/180);
      | Iq1o=InitialConditions(3)*sin(InitialConditions(6)*pi/180);
      settings: CopyFcn=powericon('psbloadfunction',gcb,'gotofrom','UpdateGotoTag');
      mask Help: web(psbhelp);
      mask StyleString: popup(3-wire Y|4-wire Y),edit,edit,edit,edit,edit,edit
      mask CallbackString: powericon('SimplifiedSynchronousMachineCback',gcb);||||||
      mask Display: plot(-60,-10,60,80,circl1,circl2,a1,a2,b1,b2,c1,c2);disp('\nSSM');color('blue');plot([0,0,40],[50,68,68]);plot([-35,-25],[50,40]);plot([-45,-35],[0,0])
  Steam Turbine and Governor : Subsystem  mask(Steam Turbine and Governor){gentype=Tandem-compound (multi-mass), reg1=[ 1  0.05    0 ], reg2=[ 0.001  0.15 ], reg3=[ -0.1  0.1  0  4.496 ], turb1=[ 0  10   3.3   0.5   ], turb2=[   0   0.36    0.36   0.28   ], HA=[ 0.046  1.430  1.465   0.192 ], KA=[ 90.44  53.88  64.59   62.94  ], DA=[ 0.0115  0.3575  0.3663   0.0137  ], ini1=250.35/555, ini2=[ 250.35/555   -51.2424   ]}
      mask prompts: gentype "Generator type"; reg1 "Regulator gain, perm. droop, dead zone [ Kp  Rp(p.u.)  Dz(p.u.) ]:"; reg2 "Speed relay and servo-motor time constants [ Tsr  Tsm ] (s):"; reg3 "Gate opening limits [ vgmin,vgmax (p.u./s)  gmin,gmax (p.u.)]:"; turb1 "Steam turbine time constants [ T2  T3  T4  T5 ] (s):"; turb2 "Turbine torque fractions [ F2  F3  F4  F5 ]:"; HA "Coeff. of inertia [ H2  H3  H4  H5 ] (s):"; KA "Stiffness coeff. [ K12  K23  K34  K45 ] (pu/rad):"; DA "Damping factors [ D2  D3  D4  D5 ] (p.u. T/p.u. dw):"; ini1 "Initial power Pm0 (p.u.):"; ini2 "Initial power and generator rotor angle [ Pm0 (p.u.)  th0(deg) ]:"
      mask help:
      | Implements a complete tandem-compound steam prime mover system, including
      | speed regulator, steam turbine and a shaft with up to 4 masses. The genererator's
      | mass is labelled mass #1 and is not included here. The shaft mass closest to the
      | generator is #2, the farthest is #5. If a mass is not to be included, set it's inertia H to
      | zero. The damping factor and rigidity coefficients corresponding to omitted masses
      | are not considered and can be left as is. When masses are omitted, the remaining
      | system is "compressed" towards the generator i.e. if only 2 masses are used, it will
      | be masses #2 and #3. The input data for the masses considered is shifted accordingly.
      mask init:
      | if gentype==1, HA=[];DA=[];KA=[]; ini2=[]; end
      | 
      | [q0,FA,Ha,Ka,Da,dtha,t,errorFlag,ctrl1,sel,massNumber] = powericon(...
      | 'STG Model',gentype,reg1,reg2,reg3,turb1,turb2,HA,KA,DA,ini1,ini2);
      | 
      | switch errorFlag
      | case 1, error('Torque fractions total (gen.A)  is not 1 p.u.');
      | case 3
      |     mess=['You requested the multi-mass shaft but set all mass inertia',...
      |         ' constants to zero. Please use the single-mass option.'];
      |     error(mess);
      | case 4
      |    mess=['Inconsistent mass inertias and power fractions. Mass #',...
      |             num2str(massNumber),' has inertia set to zero but the ',...
      |             'corresponding torque fraction is not zero.'];
      |     error(mess);
      | case 5
      |         error('Parameters error');
      | end
      mask Help: web(psbhelp);
      mask StyleString: popup(Tandem-compound (single mass)|Tandem-compound (multi-mass)),edit,edit,edit,edit,edit,edit,edit,edit,edit,edit
      mask CallbackString: powericon('psbcallbacks',gcbh,'SteamTurbine');||||||||||
      mask Display: plot([0 0],[t t])
  Synchronous Machine SI Fundamental : Subsystem  mask(Synchronous Machine){PresetModel=No, ShowDetailedParameters=on, RotorType=Salient-pole, NominalParameters=[ 187E6  13800   60   1087 ], Stator=[ 2.9069E-03  3.0892E-04  3.2164E-03  9.7153E-04 ], Field=[ 5.9013E-04  3.0712E-04 ], Dampers2=[ 0.0664, 1.387e-3, 0.0292, 6.896e-4, 7.907e-3, 2.477e-3], Dampers1=[ 1.1900E-02  4.9076E-04  2.0081E-02  1.0365E-03 ], Mechanical=[ 3.895e6 0  20 ], InitialConditions=[ 0  0  0  0  0  0  0  0  70.3192 ], SetSaturation=off, Saturation=[695.64,774.7,917.5,1001.6,1082.2,1175.9,1293.6,1430.2,1583.7;9660,10623,12243,13063,13757,14437,15180,15890,16567], DisplayVfd=off, Units=1, LoadFlowParameters=[1,0,0,0,0]}
      mask prompts: PresetModel "Preset  model"; ShowDetailedParameters "-----------------  Show detailed parameters -----------------"; RotorType "Rotor type:"; NominalParameters "Nom. power, volt., freq. and field cur. [ Pn(VA) Vn(Vrms) fn(Hz) ifn(A) ]:"; Stator "Stator [ Rs(ohm)  Ll,Lmd,Lmq(H) ]:"; Field "Field [ Rf'(ohm)  Llfd'(H) ]:"; Dampers2 "Dampers [ Rkd',Llkd'  Rkq1',Llkq1'  Rkq2',Llkq2'  ] (R=ohm,L=H):"; Dampers1 "Dampers [ Rkd',Llkd'  Rkq1',Llkq1'  ] (R=ohm,L=H):"; Mechanical "Inertia, friction factor and pole pairs [ J(kg.m^2)  F(N.m.s)  p() ]:"; InitialConditions "Init. cond. [ dw(%)  th(deg)  ia,ib,ic(A)  pha,phb,phc(deg)  Vf(V) ]:"; SetSaturation "Simulate saturation"; Saturation "Saturation parameters [ ifd1,ifd2,... (A) ; vt1,vt2,... (VLL rms) ]:"; DisplayVfd "Display Vfd which produces nominal Vt"; Units "iounits"; LoadFlowParameters "Load Flow Parameters"
      mask help: Implements a 3-phase synchronous machine modelled in the dq rotor reference frame. Stator windings are connected in wye to an internal neutral point. Press help for inputs and outputs description.
      mask init:
      | s1= -60;s2= -10;s3= 60;s4= 80;
      | block = gcb;
      | powericon('psbloadfunction',block,'gotofrom','Initialize');
      | %
      | switch RotorType
      | 	case 'Salient-pole'
      | 		Dampers = [Dampers1 0 inf];
      | 	case 'Round'
      | 		Dampers = Dampers2;
      | end
      | %
      | if SetSaturation==0
      | 	Saturation=[];
      | 	SetSaturation='off';
      | else
      | 	SetSaturation='on';
      | end
      | %
      | [NominalParameters,Stator,Field,Dampers,Mechanical,InitialConditions,v7,Saturation] = powericon('SynchronousMachineConvert',NominalParameters,Stator,Field,Dampers,Mechanical,InitialConditions,SetSaturation,Saturation,'1');;
      | Ts = powericon('SynchronousMachineInit',block);
      | [Rs,Ll,Lad,Laq,Rf,Llfd,Rkd,Rkq1,Rkq2,Llkd,Llkq1,Llkq2,H,F,p,dwo,tho,phido,phikdo,phifdo,phiqo,phikq1o,phikq2o,phib,Pb,Vb,Vb2,ib,ib2,Nb,N,N2,phis,a,Vfd]=powericon('SynchronousMachineParam',NominalParameters,Stator,Field,Dampers,Mechanical,InitialConditions,Saturation,0,1,1);
      | %
      | a5=a(1); 
      | a4=a(2); 
      | a3=a(3); 
      | a2=a(4); 
      | a1=a(5); 
      | a0=a(6);
      | Lmd=Stator(3); 
      | Lmq=Stator(4);
      | web_psb=NominalParameters(3)*2*pi;
      | one_third=1/3; 
      | sqrt3=sqrt(3);
      | % p.u. model :
      | Gain1 = Pb;
      | excAxis = 1;
      | 
      | % parameters specific to the phasor model :
      | 
      | % Computation of negative sequence impedance
      | % L"d= Ll +1/(1/Lmd +1/Llfd + 1/Llkd)
      | Lsecd=Stator(2)+1/(1/Stator(3)+1/Field(2)+1/Dampers(2));
      | % L"q= Ll +1/(1/Lmq +1/Llkq1 + 1/Llkq2)
      | Lsecq=Stator(2)+1/(1/Stator(4)+1/Dampers(4)+1/Dampers(6));
      | %L2=2(L"d*L"q/(L"d+L"q) (Kundur p881)
      | L2_pu=2*(Lsecd*Lsecq/(Lsecd+Lsecq));
      | % initial values of Id Iq: Idqo= mag(Ia) <( phi(Ia-)-thetao))
      | Idqo=InitialConditions(3)*exp(j*(InitialConditions(6)-InitialConditions(2))*pi/180);
      | Ido=real(Idqo); Iqo=imag(Idqo);
      settings: CopyFcn=powericon('psbloadfunction',gcb,'gotofrom','UpdateGotoTag');
      mask Help: web(psbhelp);
      mask StyleString: popup(No|01: 50Hz 400V 8.1kVA 1500RPM|02: 50Hz 400V 16kVA 1500RPM|03: 50Hz 400V 31.3kVA 1500RPM|04: 50Hz 400V 42.5kVA 1500RPM|05: 50Hz 400V 60kVA 1500RPM|06: 50Hz 400V 85kVA 1500RPM|07: 50Hz 400V 250kVA 1500RPM|08: 50Hz 400V 325kVA 1500RPM|09: 50Hz 400V 670kVA 1500RPM|10: 50Hz 400V 910kVA 1500RPM|11: 50Hz 400V 1320kVA 1500RPM|12: 50Hz 400V 2000kVA 1500RPM|13: 60Hz 460V 10.2kVA 1800RPM|14: 60Hz 460V 20kVA 1800RPM|15: 60Hz 460V 37.5kVA 1800RPM|16: 60Hz 460V 52.5kVA 1800RPM|17: 60Hz 460V 72.5kVA 1800RPM|18: 60Hz 460V 100kVA 1800RPM|19: 60Hz 460V 300kVA 1800RPM|20: 60Hz 460V 406kVA 1800RPM|21: 60Hz 460V 800kVA 1800RPM|22: 60Hz 460V 1075kVA 1800RPM|23: 60Hz 460V 1588kVA 1800RPM|24: 60Hz 460V 2500kVA 1800RPM),checkbox,popup(Salient-pole|Round),edit,edit,edit,edit,edit,edit,edit,checkbox,edit,checkbox,edit,edit
      mask CallbackString: powericon('SynchronousMachineCback',gcb,'FUN_SI');|powericon('SynchronousMachineCback',gcb);|powericon('SynchronousMachineCback',gcb);||||||||powericon('SynchronousMachineCback',gcb);||powericon('SynchronousMachineVfd',gcb);||
      mask Display:
      | plot(s1,s2,s3,s4,
      | [0,9,18,24,29,30,29,24,18,9,0,-9,-18,-24,-29,-30,-29,-24,-18,-9,0]*1.2,
      | [30,29,24,18,9,0,-9,-18,-24,-29,-30,-29,-24,-18,-9,0,9,18,24,29,30]*1.2+15,
      | [23,48],[27,27]+15,[36,48],[15,15],[23,48],[-27,-27]+15,
      | [0,-9,-18,-24,-16,-16,-24,-18,-9,0,9,18,24,16,16,24,18,9,0],
      | [-30,-29,-24,-18,-18,18,18,24,29,30,29,24,18,18,-18,-18,-24,-29,-30]+15);
      | color('blue');
      | plot([0,0,40],[50,68,68])
      | plot([-35,-25],[50,40])
  Synchronous Machine pu Fundamental : Subsystem  mask(Synchronous Machine){PresetModel=No, ShowDetailedParameters=on, RotorType=Salient-pole, NominalParameters=[ 187E6  13800   60], Stator=[ 2.85E-03  0.114  1.19  0.36 ], Field=[ 5.79E-04  0.114], Dampers2=[0.0652, 0.5134, 0.0287, 0.2553, 7.765e-3, 0.9167 ], Dampers1=[ 1.17E-02  0.182  1.97E-02  0384 ], Mechanical=[ 3.7 0  20 ], InitialConditions=[ 0  0  0  0  0  0  0  0  1 ], SetSaturation=off, Saturation=[0.6404,0.7127,0.8441,0.9214,0.9956,1.082,1.19,1.316,1.457;0.7,0.7698,0.8872,0.9466,0.9969,1.046,1.1,1.151,1.201], Units=0, LoadFlowParameters=[1,0,0,0,0]}
      mask prompts: PresetModel "Preset  model"; ShowDetailedParameters "-----------------  Show detailed parameters -----------------"; RotorType "Rotor type:"; NominalParameters "Nom. power, L-L volt. and freq. [ Pn(VA)  Vn(Vrms)  fn(Hz) ]:"; Stator "Stator [ Rs  Ll  Lmd  Lmq ] (pu):"; Field "Field [ Rf  Llfd ] (pu):"; Dampers2 "Dampers [ Rkd,Llkd  Rkq1,Llkq1 Rkq2,Llkq2 ] (pu):"; Dampers1 "Dampers [ Rkd,Llkd  Rkq1,Llkq1 ] (pu):"; Mechanical "Coeff. of inertia, friction factor and pole pairs [ H(s)  F(pu)  p() ]:"; InitialConditions "Init. cond. [ dw(%)  th(deg)  ia,ib,ic(pu)  pha,phb,phc(deg)  Vf(pu) ]:"; SetSaturation "Simulate saturation"; Saturation "Saturation parameters [ ifd1,ifd2,... (p.u.) ; vt1,vt2,... (p.u.) ]:"; Units "iounits"; LoadFlowParameters "Load Flow Parameters"
      mask help: Implements a 3-phase synchronous machine modelled in the dq rotor reference frame. Stator windings are connected in wye to an internal neutral point.
      mask init:
      | s1= -60;s2= -10;s3= 60;s4= 80;
      | block = gcb;
      | switch RotorType
      | 	case 'Salient-pole', 
      | 		Dampers = [Dampers1 0 inf];
      | 	case 'Round',
      | 		Dampers = Dampers2;
      | end
      | Ts = powericon('SynchronousMachineInit',block);
      | powericon('psbloadfunction',block,'gotofrom','Initialize');
      | %
      | if SetSaturation==0
      | 	Saturation=[];
      | end
      | %
      | [Rs,Ll,Lad,Laq,Rf,Llfd,Rkd,Rkq1,Rkq2,Llkd,Llkq1,Llkq2,H,F,p,dwo,tho,phido,phikdo,phifdo,phiqo,phikq1o,phikq2o,phib,Pb,Vb,Vb2,ib,ib2,Nb,N,N2,phis,a,Vfd]=powericon('SynchronousMachineParam',NominalParameters,Stator,Field,Dampers,Mechanical,InitialConditions,Saturation,0,0,1);
      | a5=a(1); 
      | a4=a(2); 
      | a3=a(3); 
      | a2=a(4); 
      | a1=a(5); 
      | a0=a(6);
      | Lmd=Stator(3); 
      | Lmq=Stator(4);
      | web_psb=NominalParameters(3)*2*pi;
      | one_third=1/3; 
      | sqrt3=sqrt(3);
      | % p.u. model :
      | Gain1 = 1;
      | excAxis = 1;
      | 
      | % parameters specific to the phasor model :
      | 
      | % Computation of negative sequence impedance
      | % L"d= Ll +1/(1/Lmd +1/Llfd + 1/Llkd)
      | Lsecd=Stator(2)+1/(1/Stator(3)+1/Field(2)+1/Dampers(2));
      | % L"q= Ll +1/(1/Lmq +1/Llkq1 + 1/Llkq2)
      | Lsecq=Stator(2)+1/(1/Stator(4)+1/Dampers(4)+1/Dampers(6));
      | %L2=2(L"d*L"q/(L"d+L"q) (Kundur p881)
      | L2_pu=2*(Lsecd*Lsecq/(Lsecd+Lsecq));
      | % initial values of Id Iq: Idqo= mag(Ia) <( phi(Ia-)-thetao))
      | Idqo=InitialConditions(3)*exp(j*(InitialConditions(6)-InitialConditions(2))*pi/180);
      | Ido=real(Idqo); Iqo=imag(Idqo);
      settings: CopyFcn=powericon('psbloadfunction',gcb,'gotofrom','UpdateGotoTag');
      mask Help: web(psbhelp);
      mask StyleString: popup(No|01: 50Hz 400V 8.1kVA 1500RPM|02: 50Hz 400V 16kVA 1500RPM|03: 50Hz 400V 31.3kVA 1500RPM|04: 50Hz 400V 42.5kVA 1500RPM|05: 50Hz 400V 60kVA 1500RPM|06: 50Hz 400V 85kVA 1500RPM|07: 50Hz 400V 250kVA 1500RPM|08: 50Hz 400V 325kVA 1500RPM|09: 50Hz 400V 670kVA 1500RPM|10: 50Hz 400V 910kVA 1500RPM|11: 50Hz 400V 1320kVA 1500RPM|12: 50Hz 400V 2000kVA 1500RPM|13: 60Hz 460V 10.2kVA 1800RPM|14: 60Hz 460V 20kVA 1800RPM|15: 60Hz 460V 37.5kVA 1800RPM|16: 60Hz 460V 52.5kVA 1800RPM|17: 60Hz 460V 72.5kVA 1800RPM|18: 60Hz 460V 100kVA 1800RPM|19: 60Hz 460V 300kVA 1800RPM|20: 60Hz 460V 406kVA 1800RPM|21: 60Hz 460V 800kVA 1800RPM|22: 60Hz 460V 1075kVA 1800RPM|23: 60Hz 460V 1588kVA 1800RPM|24: 60Hz 460V 2500kVA 1800RPM),checkbox,popup(Salient-pole|Round),edit,edit,edit,edit,edit,edit,edit,checkbox,edit,edit,edit
      mask CallbackString: powericon('SynchronousMachineCback',gcb,'FUN_PU');|powericon('SynchronousMachineCback',gcb);|powericon('SynchronousMachineCback',gcb);||||||||powericon('SynchronousMachineCback',gcb);|||
      mask Display:
      | plot(s1,s2,s3,s4,
      | [0,9,18,24,29,30,29,24,18,9,0,-9,-18,-24,-29,-30,-29,-24,-18,-9,0]*1.2,
      | [30,29,24,18,9,0,-9,-18,-24,-29,-30,-29,-24,-18,-9,0,9,18,24,29,30]*1.2+15,
      | [23,48],[27,27]+15,[36,48],[15,15],[23,48],[-27,-27]+15,
      | [0,-9,-18,-24,-16,-16,-24,-18,-9,0,9,18,24,16,16,24,18,9,0],
      | [-30,-29,-24,-18,-18,18,18,24,29,30,29,24,18,18,-18,-18,-24,-29,-30]+15);
      | color('blue');
      | plot([0,0,40],[50,68,68])
      | plot([-35,-25],[50,40])
  Synchronous Machine pu Standard : Subsystem  mask(Synchronous Machine){PresetModel=No, ShowDetailedParameters=on, RotorType=Salient-pole, NominalParameters=[ 187E6  13800   60], Reactances1=[ 1.81, 0.3, 0.23, 1.76, 0.65, 0.25, 0.15 ], Reactances2=[ 1.305, 0.296, 0.252, 0.474,  0.243,  0.18 ], dAxisTimeConstants=Open-circuit, qAxisTimeConstants=Short-circuit, TimeConstants1=[ 4.4849  0.0681  0.1  ], TimeConstants2=[ 8.0, 0.03, 1.0, 0.07 ], TimeConstants3=[  4.49  0.0681  0.0513  ], TimeConstants4=[ 8.0, 0.03, 0.3371, 0.0295 ], TimeConstants5=[ 1.01, 0.053, 0.1 ], TimeConstants6=[ 1.3201, 0.023, 1.0, 0.07 ], TimeConstants7=[  1.01  0.053  0.051266  ], TimeConstants8=[ 1.3201, 0.0231, 0.3371, 0.0295 ], StatorResistance=0.003, Mechanical=[ 3.7 0  20 ], InitialConditions=[ 0  0  0  0  0  0  0  0  1 ], SetSaturation=off, Saturation=[0.6404,0.7127,0.8441,0.9214,0.9956,1.082,1.19,1.316,1.457;0.7,0.7698,0.8872,0.9466,0.9969,1.046,1.1,1.151,1.201], Units=0.5, LoadFlowParameters=[1,0,0,0,0]}
      mask prompts: PresetModel "Preset  model"; ShowDetailedParameters "-----------------  Show detailed parameters -----------------"; RotorType "Rotor type:"; NominalParameters "Nom. power, L-L volt. and freq. [ Pn(VA)  Vn(Vrms)  fn(Hz) ]:"; Reactances1 "Reactances [ Xd Xd' Xd'' Xq Xq'  Xq'' Xl ] (pu):"; Reactances2 "Reactances [ Xd Xd' Xd'' Xq Xq'' Xl ] (pu):"; dAxisTimeConstants "d axis time constants:"; qAxisTimeConstants "q axis time constant(s):"; TimeConstants1 "Time constants [ Tdo'  Tdo''  Tqo'' ] (s):"; TimeConstants2 "Time constants [ Tdo'  Tdo''  Tqo'  Tqo'' ] (s):"; TimeConstants3 "Time constants [ Tdo'  Tdo''  Tq'' ] (s):"; TimeConstants4 "Time constants [ Tdo'  Tdo''  Tq'  Tq'' ] (s):"; TimeConstants5 "Time constants [ Td'  Td''  Tqo'' ] (s):"; TimeConstants6 "Time constants [ Td'  Td''  Tqo'  Tqo'' ] (s):"; TimeConstants7 "Time constants [ Td'  Td''  Tq'' ] (s):"; TimeConstants8 "Time constants [ Td'  Td''  Tq'  Tq'' ] (s):"; StatorResistance "Stator resistance Rs (p.u.):"; Mechanical "Coeff. of inertia, friction factor and pole pairs [ H(s)  F(pu)  p() ]:"; InitialConditions "Init. cond. [ dw(%)  th(deg)  ia,ib,ic(pu)  pha,phb,phc(deg)  Vf(pu) ]:"; SetSaturation "Simulate saturation"; Saturation "Saturation parameters [ ifd1,ifd2,... (p.u.) ; vt1,vt2,... (p.u.) ]:"; Units "iounits"; LoadFlowParameters "Load Flow Parameters"
      mask help: Implements a 3-phase synchronous machine modelled in the dq rotor reference frame. Stator windings are connected in wye to an internal neutral point.
      mask init:
      | s1= -60;s2= -10;s3= 60;s4= 80;
      | block = gcb;
      | powericon('psbloadfunction',block,'gotofrom','Initialize');
      | %
      | sit = strcmp(RotorType,'Round') + strcmp(qAxisTimeConstants,'Short-circuit')*2 + strcmp(dAxisTimeConstants,'Short-circuit')*4;
      | switch sit
      |     case 0, line2 = Reactances2; line3 = TimeConstants1;
      |     case 1, line2 = Reactances1; line3 = TimeConstants2;
      |     case 2, line2 = Reactances2; line3 = TimeConstants3;
      |     case 3, line2 = Reactances1; line3 = TimeConstants4;
      |     case 4, line2 = Reactances2; line3 = TimeConstants5;
      |     case 5, line2 = Reactances1; line3 = TimeConstants6;
      |     case 6, line2 = Reactances2; line3 = TimeConstants7;
      |     case 7, line2 = Reactances1; line3 = TimeConstants8;
      | end
      | %
      | if SetSaturation==0
      | 	Saturation=[];
      | 	SetSaturation='off';
      | else
      | 	SetSaturation='on';
      | end
      | %
      | [NominalParameters,Stator,Field,Dampers,Mechanical,InitialConditions,v7,Saturation] = powericon('SynchronousMachineConvert',NominalParameters,line2,line3,StatorResistance,Mechanical,InitialConditions,SetSaturation,Saturation,'3',sit,block);
      | Ts = powericon('SynchronousMachineInit',block);
      | [Rs,Ll,Lad,Laq,Rf,Llfd,Rkd,Rkq1,Rkq2,Llkd,Llkq1,Llkq2,H,F,p,dwo,tho,phido,phikdo,phifdo,phiqo,phikq1o,phikq2o,phib,Pb,Vb,Vb2,ib,ib2,Nb,N,N2,phis,a,Vfd]=powericon('SynchronousMachineParam',NominalParameters,Stator,Field,Dampers,Mechanical,InitialConditions,Saturation,0,0,1);
      | %
      | a5=a(1); 
      | a4=a(2); 
      | a3=a(3); 
      | a2=a(4); 
      | a1=a(5); 
      | a0=a(6);
      | Lmd=Stator(3); 
      | Lmq=Stator(4);
      | web_psb=NominalParameters(3)*2*pi;
      | one_third=1/3; 
      | sqrt3=sqrt(3);
      | % p.u. model :
      | Gain1 = 1;
      | excAxis = 1;
      | 
      | % parameters specific to the phasor model :
      | 
      | % Computation of negative sequence impedance
      | % L"d= Ll +1/(1/Lmd +1/Llfd + 1/Llkd)
      | Lsecd=Stator(2)+1/(1/Stator(3)+1/Field(2)+1/Dampers(2));
      | % L"q= Ll +1/(1/Lmq +1/Llkq1 + 1/Llkq2)
      | Lsecq=Stator(2)+1/(1/Stator(4)+1/Dampers(4)+1/Dampers(6));
      | %L2=2(L"d*L"q/(L"d+L"q) (Kundur p881)
      | L2_pu=2*(Lsecd*Lsecq/(Lsecd+Lsecq));
      | % initial values of Id Iq: Idqo= mag(Ia) <( phi(Ia-)-thetao))
      | Idqo=InitialConditions(3)*exp(j*(InitialConditions(6)-InitialConditions(2))*pi/180);
      | Ido=real(Idqo); Iqo=imag(Idqo);
      settings: CopyFcn=powericon('psbloadfunction',gcb,'gotofrom','UpdateGotoTag');
      mask Help: web(psbhelp);
      mask StyleString: popup(No|01: 50Hz 400V 8.1kVA 1500RPM|02: 50Hz 400V 16kVA 1500RPM|03: 50Hz 400V 31.3kVA 1500RPM|04: 50Hz 400V 42.5kVA 1500RPM|05: 50Hz 400V 60kVA 1500RPM|06: 50Hz 400V 85kVA 1500RPM|07: 50Hz 400V 250kVA 1500RPM|08: 50Hz 400V 325kVA 1500RPM|09: 50Hz 400V 670kVA 1500RPM|10: 50Hz 400V 910kVA 1500RPM|11: 50Hz 400V 1320kVA 1500RPM|12: 50Hz 400V 2000kVA 1500RPM|13: 60Hz 460V 10.2kVA 1800RPM|14: 60Hz 460V 20kVA 1800RPM|15: 60Hz 460V 37.5kVA 1800RPM|16: 60Hz 460V 52.5kVA 1800RPM|17: 60Hz 460V 72.5kVA 1800RPM|18: 60Hz 460V 100kVA 1800RPM|19: 60Hz 460V 300kVA 1800RPM|20: 60Hz 460V 406kVA 1800RPM|21: 60Hz 460V 800kVA 1800RPM|22: 60Hz 460V 1075kVA 1800RPM|23: 60Hz 460V 1588kVA 1800RPM|24: 60Hz 460V 2500kVA 1800RPM),checkbox,popup(Salient-pole|Round),edit,edit,edit,popup(Open-circuit|Short-circuit),popup(Open-circuit|Short-circuit),edit,edit,edit,edit,edit,edit,edit,edit,edit,edit,edit,checkbox,edit,edit,edit
      mask CallbackString: powericon('SynchronousMachineCback',gcb,'STD_PU');|powericon('SynchronousMachineCback',gcb);|powericon('SynchronousMachineCback',gcb);||||powericon('SynchronousMachineCback',gcb);|powericon('SynchronousMachineCback',gcb);|||powericon('SynchronousMachineCback',gcb);|||||||||powericon('SynchronousMachineCback',gcb);|||
      mask Display:
      | plot(s1,s2,s3,s4,
      | [0,9,18,24,29,30,29,24,18,9,0,-9,-18,-24,-29,-30,-29,-24,-18,-9,0]*1.2,
      | [30,29,24,18,9,0,-9,-18,-24,-29,-30,-29,-24,-18,-9,0,9,18,24,29,30]*1.2+15,
      | [23,48],[27,27]+15,[36,48],[15,15],[23,48],[-27,-27]+15,
      | [0,-9,-18,-24,-16,-16,-24,-18,-9,0,9,18,24,16,16,24,18,9,0],
      | [-30,-29,-24,-18,-18,18,18,24,29,30,29,24,18,18,-18,-18,-24,-29,-30]+15);
      | color('blue');
      | plot([0,0,40],[50,68,68])
      | plot([-35,-25],[50,40])
